simulink library "a71real"  (R2016a)
settings: Solver=ode45  StartTime=0.0  StopTime=10.0  RelTol=1e-3
values from neighbouring files (symbols this model uses):
  c_M = 1.0    (= 1)    [DCTEST.m]    (also in a71test.m)
  J_A = 2.0    (= 2)    [DCTEST.m]    (also in a71test.m)
  L_A = 0.15    [DCTEST.m]    (also in a71test.m)
  Phi = 1.5    [DCTEST.m]    (also in a71test.m)
  R_A = 2.0    (= 2)    [DCTEST.m]    (also in a71test.m)
libraries: simulink x1
settings Model: Creator=mam1205  LastModifiedBy=mam1205
settings DataIOCC: LimitDataPoints=on
settings DebuggingCC: AllowSymbolicDim=off

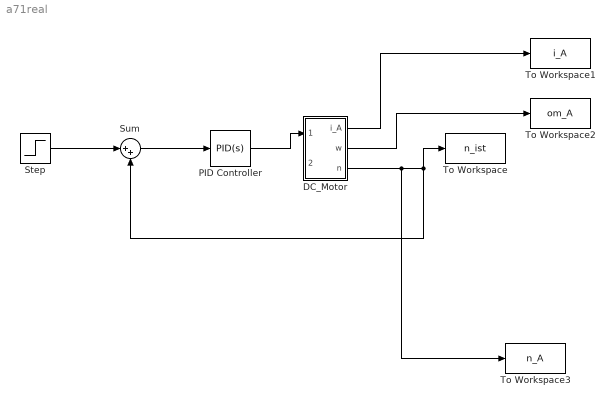
== system a71real ==
  "DC_Motor " : Subsystem
  PID Controller : simulink/Continuous/PID Controller  Controller=PID  TimeDomain=Continuous-time  SampleTime=-1  IntegratorMethod=Forward Euler  FilterMethod=Forward Euler  Form=Parallel  UseFilter=on  ControllerParametersSource=internal  P=1  I=1  D=0  N=100  InitialConditionSource=internal  InitialConditionForIntegrator=0  InitialConditionForFilter=0  ExternalReset=none  LimitOutput=off  UpperSaturationLimit=inf  LowerSaturationLimit=-inf  LinearizeAsGain=on  AntiWindupMode=none  Kb=1  TrackingMode=off  Kt=1  PParamMin=[]  PParamMax=[]  IParamMin=[]  IParamMax=[]  DParamMin=[]  DParamMax=[]  NParamMin=[]  NParamMax=[]  KbParamMin=[]  KbParamMax=[]  KtParamMin=[]  KtParamMax=[]  POutMin=[]  POutMax=[]  IOutMin=[]  IOutMax=[]  DOutMin=[]  DOutMax=[]  NOutMin=[]  NOutMax=[]  KbOutMin=[]  KbOutMax=[]  KtOutMin=[]  KtOutMax=[]  IntegratorOutMin=[]  IntegratorOutMax=[]  FilterOutMin=[]  FilterOutMax=[]  SumOutMin=[]  SumOutMax=[]  SumI1OutMin=[]  SumI1OutMax=[]  SumI2OutMin=[]  SumI2OutMax=[]  SumI3OutMin=[]  SumI3OutMax=[]  SumDOutMin=[]  SumDOutMax=[]  SaturationOutMin=[]  SaturationOutMax=[]  IntegratorContinuousStateAttributes=''  IntegratorStateMustResolveToSignalObject=off  IntegratorRTWStateStorageClass=Auto  FilterContinuousStateAttributes=''  FilterStateMustResolveToSignalObject=off  FilterRTWStateStorageClass=Auto  DifferentiatorICPrevScaledInput=0  DifferentiatorOutMin=[]  DifferentiatorOutMax=[]
  Step : Step  SampleTime=0
  Sum : Sum  Inputs=|++
  To Workspace : ToWorkspace  VariableName=n_ist  SaveFormat=Timeseries  SampleTime=-1
  To Workspace1 : ToWorkspace  VariableName=i_A  SaveFormat=Timeseries  SampleTime=-1
  To Workspace2 : ToWorkspace  VariableName=om_A  SaveFormat=Timeseries  SampleTime=-1
  To Workspace3 : ToWorkspace  VariableName=n_A  SaveFormat=Timeseries  SampleTime=-1
  wires:
  Step/1 -> Sum/1
  Sum/1 -> PID Controller/1
  "DC_Motor "/3(n) -> To Workspace/1, Sum/2, To Workspace3/1
  "DC_Motor "/1(i_A) -> To Workspace1/1
  "DC_Motor "/2(w) -> To Workspace2/1
  PID Controller/1 -> "DC_Motor "/1(u_A)

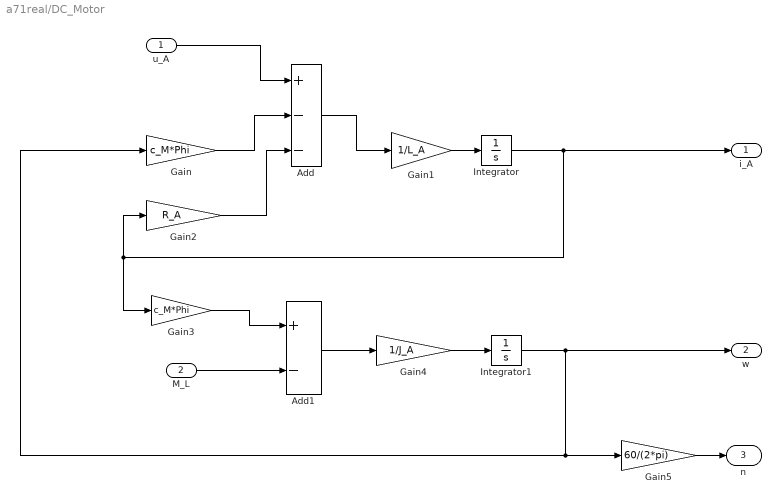
== system a71real/DC_Motor  ==
  u_A : Inport
  M_L : Inport  Port=2
  Add : Sum  Inputs=+--
  Add1 : Sum  Inputs=+-
  Gain : Gain  Gain=c_M*Phi
  Gain1 : Gain  Gain=1/L_A
  Gain2 : Gain  Gain=R_A
  Gain3 : Gain  Gain=c_M*Phi
  Gain4 : Gain  Gain=1/J_A
  Gain5 : Gain  Gain=60/(2*pi)
  Integrator : Integrator
  Integrator1 : Integrator
  i_A : Outport
  w : Outport  Port=2
  n : Outport  Port=3
  wires:
  u_A/1 -> Add/1
  Add/1 -> Gain1/1
  Gain1/1 -> Integrator/1
  Integrator/1 -> i_A/1, Gain2/1, Gain3/1
  Gain2/1 -> Add/3
  Gain3/1 -> Add1/1
  M_L/1 -> Add1/2
  Gain/1 -> Add/2
  Integrator1/1 -> w/1, Gain/1, Gain5/1
  Gain4/1 -> Integrator1/1
  Gain5/1 -> n/1
  Add1/1 -> Gain4/1
